simulink model "door_simulink_secondway"  (R2023b)
settings: Solver=VariableStepAuto  StartTime=0.0  StopTime=3  RelTol=1e-3
values from neighbouring files (symbols this model uses):
  A = plant.A    [door.m]
  B = plant.B    [door.m]
  C = [0,0,1]    [door.m]
  K = place(A,B,pc)    [door.m]
  Ntilda = rscale(plant, K)    [door.m]
settings Model: Creator=demkv  LastModifiedBy=demkv

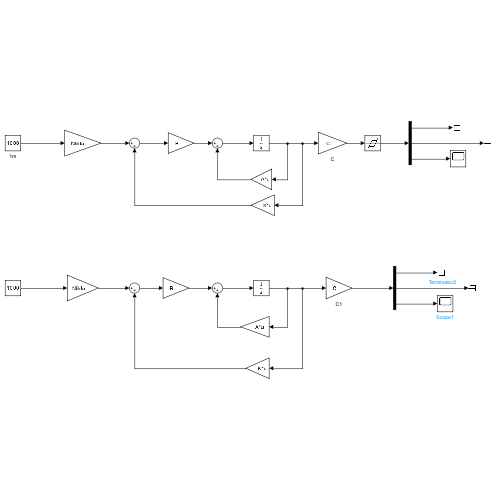
[thumbnail: Simulink's stored preview of the top-level diagram]
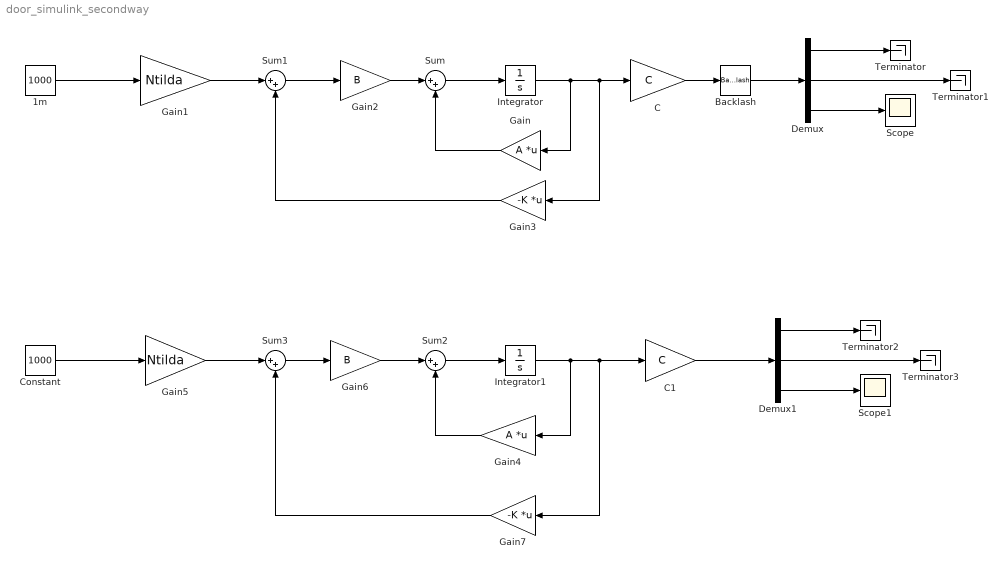
== system door_simulink_secondway ==
  1m : Constant  Value=1000
  Backlash : Backlash
  C : Gain  Gain=C
  C1 : Gain  Gain=C
  Constant : Constant  Value=1000
  Demux : Demux  Outputs=3
  Demux1 : Demux  Outputs=3
  Gain : Gain  Gain=A  Multiplication=Matrix(K*u)
  Gain1 : Gain  Gain=Ntilda
  Gain2 : Gain  Gain=B
  Gain3 : Gain  Gain=-K  Multiplication=Matrix(K*u)
  Gain4 : Gain  Gain=A  Multiplication=Matrix(K*u)
  Gain5 : Gain  Gain=Ntilda
  Gain6 : Gain  Gain=B
  Gain7 : Gain  Gain=-K  Multiplication=Matrix(K*u)
  Integrator : Integrator
  Integrator1 : Integrator
  Scope : Scope
  Scope1 : Scope
  Sum{,1..3} (4 alike) : Sum  Inputs=|++
  Terminator{,1..3} (4 alike) : Terminator
  wires:
  Gain/1 -> Sum/2
  Integrator/1 -> Gain/1, Gain3/1, C/1
  Sum/1 -> Integrator/1
  Gain2/1 -> Sum/1
  Sum1/1 -> Gain2/1
  Gain3/1 -> Sum1/2
  C/1 -> Backlash/1
  Gain1/1 -> Sum1/1
  1m/1 -> Gain1/1
  Gain4/1 -> Sum2/2
  Sum3/1 -> Gain6/1
  Gain7/1 -> Sum3/2
  Integrator1/1 -> Gain4/1, Gain7/1, C1/1
  Sum2/1 -> Integrator1/1
  Gain6/1 -> Sum2/1
  Constant/1 -> Gain5/1
  Gain5/1 -> Sum3/1
  Backlash/1 -> Demux/1
  Demux/2 -> Terminator1/1
  Demux1/2 -> Terminator3/1
  C1/1 -> Demux1/1
  Demux/1 -> Terminator/1
  Demux/3 -> Scope/1
  Demux1/1 -> Terminator2/1
  Demux1/3 -> Scope1/1
